simulink model "host_int16_2M"  (R2022b)
settings: Solver=VariableStepAuto  StartTime=0.0  StopTime=1.2  RelTol=1e-3
undefined symbols (not defined in the file): data_size, SAMPLE_TIME
libraries: instrumentseriallib x2
settings Model: Creator=Jan  LastModifiedBy=Jan
settings DataIOCC: ReturnWorkspaceOutputs=off
settings DebuggingCC: ParameterOverflowMsg=none

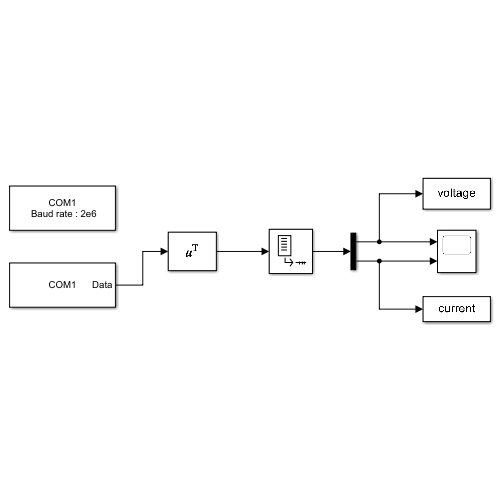
[thumbnail: Simulink's stored preview of the top-level diagram]
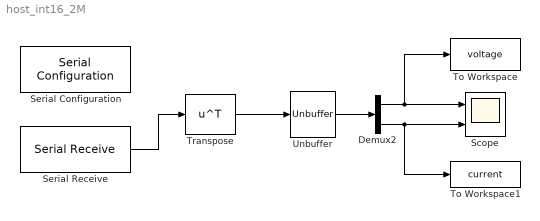
== system host_int16_2M ==
  Demux2 : Demux  Outputs=2
  Scope : Scope  NumInputPorts=2
  Serial Configuration : instrumentseriallib/Serial Configuration  Priority=-200000  PortSel=COM1  Port=COM1  ComPort=COM1  BaudRate=2e6  DataBits=8  Parity=none  StopBits=1  ByteOrder=little-endian  FlowControl=hardware  Timeout=2  SimulateUsing=Interpreted execution  BlockInModel=on  aMode=1
  Serial Receive : instrumentseriallib/Serial Receive  PortSel=COM1  Port=COM1  ComPort=COM1  DataType=int16  SaveDataType=uint8  ToggleHeader=on  Header="[ 83  83 ]"  ToggleTerminator=on  Terminator=Custom terminator  CustomTerminator="[ 69  69 ]"  InputFormat=Column major  ToggleDataSize=on  DataSize="[2  data_size]"  EnableBlockingMode=on  ActionDataUnavailable=Output last received value  ActionWhenDataUnavailable=Output last received value  CustomValue=0  SampleTime=SAMPLE_TIME*data_size  SimulateUsing=Interpreted execution  BlockInModel=on  aMode=1
  To Workspace : ToWorkspace  VariableName=voltage  SampleTime=-1
  To Workspace1 : ToWorkspace  VariableName=current  SampleTime=-1
  Transpose : Math  Operator=transpose  SignedPower=on
  Unbuffer : Unbuffer
  wires:
  Demux2/2 -> Scope/2, To Workspace1/1
  Demux2/1 -> Scope/1, To Workspace/1
  Unbuffer/1 -> Demux2/1
  Transpose/1 -> Unbuffer/1
  Serial Receive/1 -> Transpose/1
